simulink model "main040_FOPDT"  (R2023b)
settings: Solver=VariableStepAuto  StartTime=0.0  StopTime=10.0  RelTol=1e-3
settings Model: Creator=YYlab_05  LastModifiedBy=YYlab_05

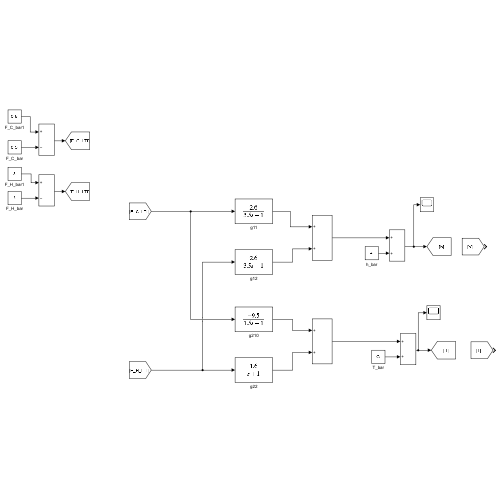
[thumbnail: Simulink's stored preview of the top-level diagram]
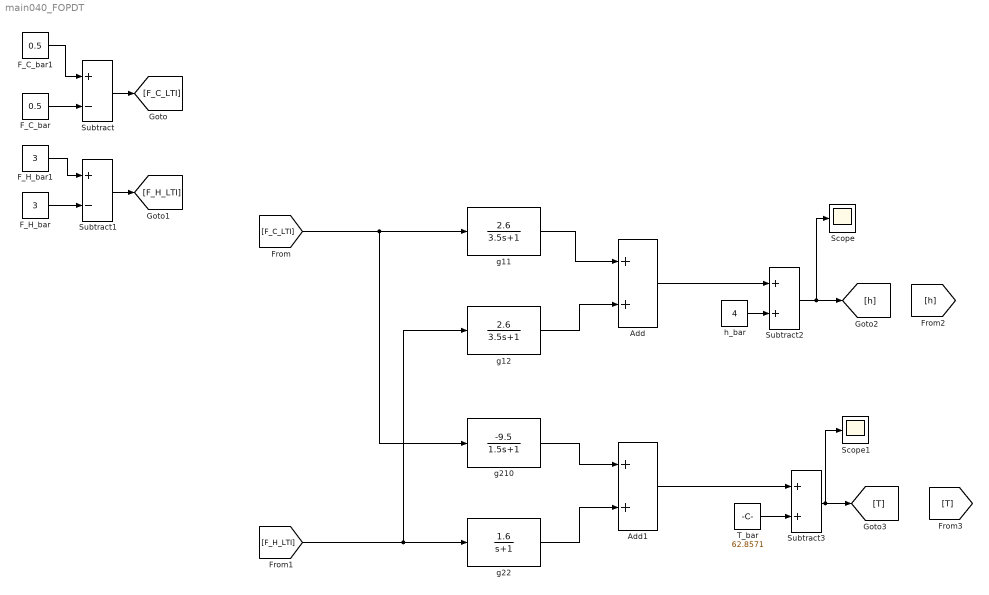
== system main040_FOPDT ==
  Add : Sum
  Add1 : Sum
  F_C_bar : Constant  Value=0.5
  F_C_bar1 : Constant  Value=0.5
  F_H_bar : Constant  Value=3
  F_H_bar1 : Constant  Value=3
  Scope : Scope
  Scope1 : Scope
  Subtract : Sum  Inputs=+-
  Subtract1 : Sum  Inputs=+-
  Subtract2 : Sum
  Subtract3 : Sum
  T_bar : Constant  Value=62.8571
  g11 : TransferFcn  Numerator=[2.6]  Denominator=[3.5 1]
  g12 : TransferFcn  Numerator=2.6  Denominator=[3.5 1]
  g210 : TransferFcn  Numerator=[-9.5]  Denominator=[1.5 1]
  g22 : TransferFcn  Numerator=1.6  Denominator=[1 1]
  h_bar : Constant  Value=4
  wires:
  [F_C_LTI] -> g11/1, g210/1
  [F_H_LTI] -> g22/1, g12/1
  g11/1 -> Add/1
  Add/1 -> Subtract2/1
  g22/1 -> Add1/2
  g12/1 -> Add/2
  g210/1 -> Add1/1
  Subtract/1 -> [F_C_LTI]
  F_C_bar/1 -> Subtract/2
  F_H_bar/1 -> Subtract1/2
  Subtract1/1 -> [F_H_LTI]
  F_C_bar1/1 -> Subtract/1
  F_H_bar1/1 -> Subtract1/1
  h_bar/1 -> Subtract2/2
  Subtract2/1 -> Scope/1, [h]
  T_bar/1 -> Subtract3/2
  Add1/1 -> Subtract3/1
  Subtract3/1 -> Scope1/1, [T]
